simulink model "Simulatore_NL"  (R2025b)
settings: Solver=VariableStepAuto  StartTime=0.0  StopTime=5.0  RelTol=1e-3
undefined symbols (not defined in the file): g_val, m_val
settings Model: Creator=david  LastModifiedBy=david

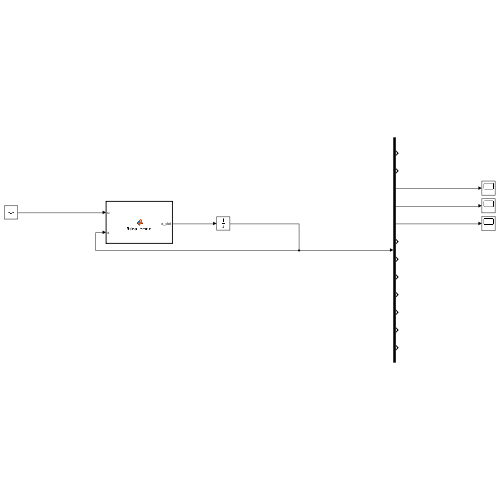
[thumbnail: Simulink's stored preview of the top-level diagram]
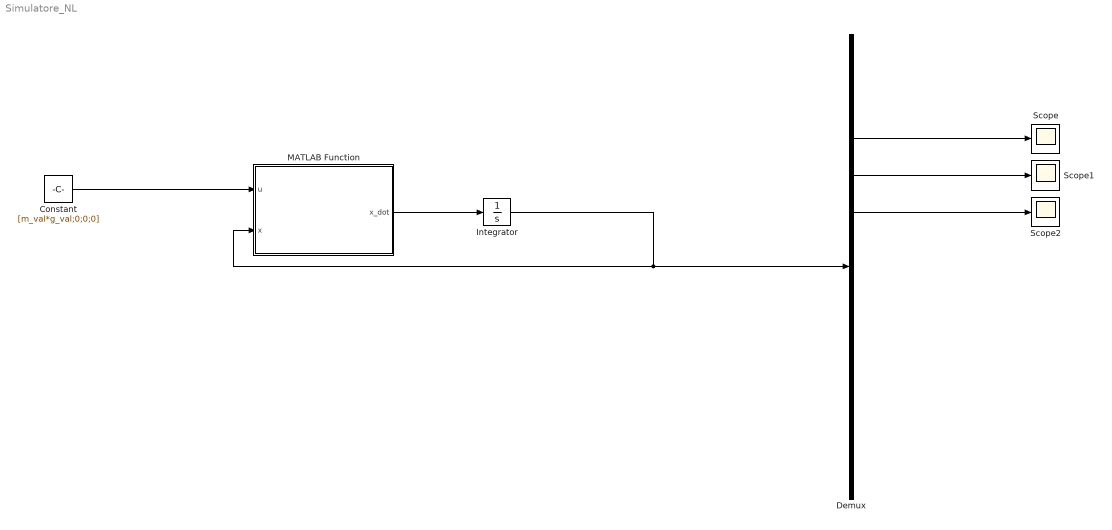
== system Simulatore_NL ==
  Constant : Constant  Value=[m_val*g_val;0;0;0]
  Demux : Demux  Outputs=12
  Integrator : Integrator  InitialCondition=[0;0;1.0;0.5;0.5;0;5.0;0;0;0;0;0]
  MATLAB Function : MATLAB Function  TreatAsAtomicUnit=on
  Scope : Scope
      settings: ActiveDisplayYMinimum=-30.708366730392147  ActiveDisplayYMaximum=4.52315185893246
  Scope1 : Scope
      settings: ActiveDisplayYMinimum=0.4  ActiveDisplayYMaximum=0.6
  Scope2 : Scope
      settings: ActiveDisplayYMinimum=0.4  ActiveDisplayYMaximum=0.6  DataLoggingVariableName=ScopeData2
  wires:
  Constant/1 -> MATLAB Function/1(u)
  MATLAB Function/1(x_dot) -> Integrator/1
  Integrator/1 -> MATLAB Function/2(x), Demux/1
  Demux/3 -> Scope/1
  Demux/4 -> Scope1/1
  Demux/5 -> Scope2/1

== matlab function Simulatore_NL/MATLAB Function ==
  data: u input; x_dot output; x input
function x_dot = fisica_drone(u, x)

    % Prende funzioni da matlab
    coder.extrinsic('drone_dynamics', 'evalin');
    
    % Inizializzazione vettore di uscita
    x_dot = zeros(12,1);
    
    % Ricavo funzioni da Workspace
    M_fun = evalin('base', 'M_fun');
    C_fun = evalin('base', 'C_fun');
    B_fun = evalin('base', 'B_fun');
    G_n   = evalin('base', 'G_n');
    

    x_dot = drone_dynamics(0, x, u, M_fun, C_fun, G_n, B_fun);
end
